simulink library "QDMS4CSD"  (R2013a)
settings: Solver=ode4  StartTime=0.0  StopTime=5  FixedStep=0.1  RelTol=1e-3
undefined symbols (not defined in the file): DiscIntNeverNeededParam, IC, quadModel
libraries: simulink x16
(part 3 of 3)

== system QDMS4CSD/Sampled Quadcopter System Components/On-board State Estimation/State Estimation and Complimentary Mixing/Subsystem/Phi_dot composer1 ==
  note: H_Phi = [1,tan(The)*sin(Phi), tan(The)*cos(Phi);
      |          0,         cos(Phi),         -sin(Phi);
      |          0,sin(Phi)/cos(The),cos(Phi)/cos(The)];
      | Phidot = H_Phi*omb_bi; %% Units OK SI
  Phi : Inport
  Theta : Inport  Port=2
  Q : Inport  Port=3
  R : Inport  Port=4
  Divide : Product  Inputs=**/
  Divide1 : Product  Inputs=**/
  Sum : Sum  Inputs=|++
  Trigonometric Function : Trigonometry  Operator=sincos
  Trigonometric Function1 : Trigonometry  Operator=cos
  psiDot : Outport
  wires:
  Sum/1 -> psiDot/1
  Phi/1 -> Trigonometric Function/1
  Trigonometric Function/1 -> Divide/2
  Theta/1 -> Trigonometric Function1/1
  Divide/1 -> Sum/1
  Trigonometric Function1/1 -> Divide/3, Divide1/3
  Q/1 -> Divide/1
  R/1 -> Divide1/2
  Divide1/1 -> Sum/2
  Trigonometric Function/2 -> Divide1/1

== system QDMS4CSD/Sampled Quadcopter System Components/On-board State Estimation/State Estimation and Complimentary Mixing/Subsystem/Theta_dot composer1 ==
  note: H_Phi = [1,tan(The)*sin(Phi), tan(The)*cos(Phi);
      |          0,         cos(Phi),         -sin(Phi);
      |          0,sin(Phi)/cos(The),cos(Phi)/cos(The)];
      | Phidot = H_Phi*omb_bi; %% Units OK SI
  Phi : Inport
  Q : Inport  Port=2
  R : Inport  Port=3
  Product : Product
  Product1 : Product
  Scope : Scope  NumInputPorts=2
      settings: YMin=-5~-5  YMax=5~5  SaveName=ScopeData6
  Sum : Sum  Inputs=|++
  Trigonometric Function2 : Trigonometry  Operator=sincos
  Unary Minus : UnaryMinus
  thetaDot : Outport
  wires:
  Sum/1 -> thetaDot/1
  Phi/1 -> Trigonometric Function2/1
  Q/1 -> Product/2
  Product/1 -> Sum/1
  Trigonometric Function2/1 -> Scope/2, Unary Minus/1
  Unary Minus/1 -> Scope/1, Product1/1
  R/1 -> Product1/2
  Product1/1 -> Sum/2
  Trigonometric Function2/2 -> Product/1

== system QDMS4CSD/Sampled Quadcopter System Components/On-board State Estimation/State Estimation and Complimentary Mixing/Subsystem1/Magnitude ==
  x_acc : Inport
  y_acc : Inport  Port=2
  z_acc : Inport  Port=3
  Demux1 : Demux  Outputs=3
  Math Function : Math  Operator=square  SaturateOnIntegerOverflow=on
  Mux : Mux  Inputs=3
  Sqrt : Sqrt  SaturateOnIntegerOverflow=on
  Sum : Sum  Inputs=+++
  |g| : Outport
  wires:
  Sqrt/1 -> |g|/1  "mag_acc"
  Sum/1 -> Sqrt/1
  Demux1/3 -> Sum/3
  Mux/1 -> Math Function/1
  Math Function/1 -> Demux1/1
  Demux1/1 -> Sum/1
  Demux1/2 -> Sum/2
  y_acc/1 -> Mux/2
  x_acc/1 -> Mux/1
  z_acc/1 -> Mux/3

== system QDMS4CSD/Sampled Quadcopter System Components/On-board State Estimation/getMotion6()/Accelerometer/Raw Data Scaling ==
  In1 : Inport
  Data Type Conversion : DataTypeConversion  OutDataTypeStr=int16  SaturateOnIntegerOverflow=on
  Gain1 : Gain  Gain=-16384  RndMeth=Round  SaturateOnIntegerOverflow=on
  Out1 : Outport
  wires:
  Gain1/1 -> Data Type Conversion/1
  In1/1 -> Gain1/1
  Data Type Conversion/1 -> Out1/1

== system QDMS4CSD/Sampled Quadcopter System Components/On-board State Estimation/getMotion6()/Accelerometer/Raw Data Scaling1 ==
  In1 : Inport
  Data Type Conversion : DataTypeConversion  OutDataTypeStr=int16
  Gain1 : Gain  Gain=16384  RndMeth=Round  SaturateOnIntegerOverflow=on
  Out1 : Outport
  wires:
  Gain1/1 -> Data Type Conversion/1
  In1/1 -> Gain1/1
  Data Type Conversion/1 -> Out1/1

== system QDMS4CSD/Sampled Quadcopter System Components/On-board State Estimation/getMotion6()/Accelerometer/Raw Data Scaling2 ==
  In1 : Inport
  Data Type Conversion : DataTypeConversion  OutDataTypeStr=int16
  Gain1 : Gain  Gain=16384  RndMeth=Round  SaturateOnIntegerOverflow=on
  Out1 : Outport
  wires:
  Gain1/1 -> Data Type Conversion/1
  In1/1 -> Gain1/1
  Data Type Conversion/1 -> Out1/1

== system QDMS4CSD/Sampled Quadcopter System Components/On-board State Estimation/getMotion6()/Gyro signals/Gyro Raw Data Scaling ==
  In1 : Inport
  Data Type Conversion : DataTypeConversion  OutDataTypeStr=int16  SaturateOnIntegerOverflow=on
  Gain1 : Gain  Gain=180*131.1/pi  RndMeth=Round  SaturateOnIntegerOverflow=on
  Out1 : Outport
  wires:
  Gain1/1 -> Data Type Conversion/1
  In1/1 -> Gain1/1
  Data Type Conversion/1 -> Out1/1

== system QDMS4CSD/Sampled Quadcopter System Components/On-board State Estimation/getMotion6()/Gyro signals/Gyro Raw Data Scaling1 ==
  In1 : Inport
  Data Type Conversion : DataTypeConversion  OutDataTypeStr=int16  SaturateOnIntegerOverflow=on
  Gain1 : Gain  Gain=180*131.1/pi  RndMeth=Round  SaturateOnIntegerOverflow=on
  Out1 : Outport
  wires:
  Gain1/1 -> Data Type Conversion/1
  In1/1 -> Gain1/1
  Data Type Conversion/1 -> Out1/1

== system QDMS4CSD/Sampled Quadcopter System Components/On-board State Estimation/getMotion6()/Gyro signals/Gyro Raw Data Scaling2 ==
  In1 : Inport
  Data Type Conversion : DataTypeConversion  OutDataTypeStr=int16  SaturateOnIntegerOverflow=on
  Gain1 : Gain  Gain=180*131.1/pi  RndMeth=Round  SaturateOnIntegerOverflow=on
  Out1 : Outport
  wires:
  Gain1/1 -> Data Type Conversion/1
  In1/1 -> Gain1/1
  Data Type Conversion/1 -> Out1/1
